simulink model "gm_model2"  (R2019b)
settings: Solver=FixedStepDiscrete  StartTime=0.0  StopTime=0.001  FixedStep=1e-9  RelTol=1e-3
settings Model: Creator=bwieczorek  LastModifiedBy=bwieczorek
settings OptimizationCC: BlockReduction=off  ConditionallyExecuteInputs=off
settings DebuggingCC: InheritedTsInSrcMsg=none

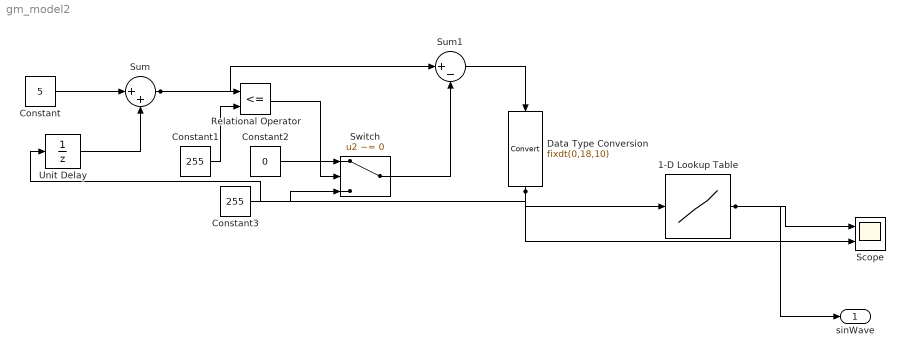
== system gm_model2 ==
  1-D Lookup Table : Lookup_n-D  NumberOfTableDimensions=1  BreakpointsSpecification=Even spacing  BreakpointsForDimension1=[linspace(0, 255, 256)]  BreakpointsForDimension1FirstPoint=0  BreakpointsForDimension1DataTypeStr=fixdt(0,18, 10)  IndexSearchMethod=Linear search  BeginIndexSearchUsingPreviousIndexResult=on  Table=sin([0:0.024639:2*3.141592])  TableDataTypeStr=fixdt(1,18,17)  ExtrapMethod=Clip  RemoveProtectionInput=on  UseLastTableValue=on  InternalRulePriority=Speed  OutDataTypeStr=fixdt(1,18,17)  RndMeth=Simplest  SupportTunableTableSize=on  MaximumIndicesForEachDimension=[255]  InputSameDT=on
  Constant : Constant  Value=5  OutDataTypeStr=fixdt(0,18,10)  SampleTime=1e-6
  Constant1 : Constant  Value=255  OutDataTypeStr=fixdt(0,18,10)  SampleTime=1e-6  LockScale=on
  Constant2 : Constant  Value=0  OutDataTypeStr=fixdt(0,18,10)  SampleTime=1e-6
  Constant3 : Constant  Value=255  OutDataTypeStr=fixdt(0,18,10)  SampleTime=1e-6
  Data Type Conversion : DataTypeConversion  OutDataTypeStr=fixdt(0,18,10)
  Relational Operator : RelationalOperator  Operator=<=  OutDataTypeStr=boolean  RndMeth=Nearest
  Scope : Scope  NumInputPorts=2
  Sum : Sum  Inputs=|++
  Sum1 : Sum  Inputs=|+-
  Switch : Switch  Criteria=u2 ~= 0
  Unit Delay : UnitDelay  SampleTime=-1  HasFrameUpgradeWarning=on
  "sinWave " : Outport  VectorParamsAs1DForOutWhenUnconnected=off
  wires:
  1-D Lookup Table/1 -> Scope/1, "sinWave "/1
  Constant/1 -> Sum/1
  Constant1/1 -> Relational Operator/2
  Constant2/1 -> Switch/1
  Constant3/1 -> Switch/3
  Data Type Conversion/1 -> 1-D Lookup Table/1, Unit Delay/1, Scope/2
  Relational Operator/1 -> Switch/2
  Sum/1 -> Sum1/1, Relational Operator/1
  Sum1/1 -> Data Type Conversion/1
  Switch/1 -> Sum1/2
  Unit Delay/1 -> Sum/2
